simulink model "batteryModuleDoc_example"  (R2023a)
settings: Solver=ode23t  StartTime=0.0  StopTime=900  MaxStep=0.05  RelTol=1e-3  AbsTol=1e-3
InitFcn:
  | % Parameters
  | battery_vecT=[273.15, 298.15, 323.15]; % [K]
  | battery_vecAhr=5*[2.9, 4.1, 4.2];        % [Ahr]
  | battery_vecSOC=[0, .25, .75, 1];       % [-]
  | %
  | battery_V0=[3.20, 3.10, 3.14; ...
  |             3.25, 3.27, 3.30;...
  |             3.28, 3.31, 3.34;...
  |             3.33, 3.50, 3.59];         % No-load voltage, V0(SOC,T)
  | battery_R0=2*[.030, .015, .002; ...
  |             .040, .017, .008; ...
  |             .039, .012, .006; ...
  |             .027, .013, .021];         % Terminal resistance, R0(SOC,T)
  | battery_R1=[.089, .076, .010; ...
  |             .042, .022, .099; ...
  |             .019, .007, .002; ...
  |             .051, .043, .029];         % First polarization resistance, R1(SOC,T)
  | battery_Tau1=[44, 148, 235; ...
  |               93, 110, 1000; ...
  |               19, 27, 133; ...
  |               .5, 22, 3];              % First time constant, tau1(SOC,T)
  | battery_R2=[.014, .382, .407; ...
  |             .028, .006, .007; ...
  |             .014, .007, .006; ...
  |             .333, .956, .912];         % Second polarization resistance, R2(SOC,T)
  | battery_Tau2=[1, 44, 5644; ...
  |               11, 24, 506; ...
  |               2, 14, 330; ...
  |               3310, 13419, 30216];     % Second time constant, tau2(SOC,T)
  | 
  | %% Battery Module : Cell Thermal
  | battery_thermalMass=500;               % Battery cell thermal mass
  | battery_thermalK_thru=0.8;             % Battery cell through-plane thermal conductivity
  | battery_thermalK_in=20;                % Battery cell in-plane thermal conductivity
  | 
  | %% Battery Module : Module Electrical
  | battery_Np=2;
  | battery_Ns=15;
  | battery_cellH=0.65;
  | battery_cellW=0.20;
  | battery_cellT=0.02;
  | battery_extR=0.001;
  | 
  | %% Battery Module : Module Thermal
  | battery_sidesHTC=1;
  | battery_extHeat=zeros(1,battery_Np*battery_Ns);
  | 
  | %% Battery Module : Cell-to-Cell Variation
  | battery_iniT=ambientTemp*ones(1,battery_Np*battery_Ns);
  | battery_iniSOC=initialSOCvalue*ones(1,battery_Np*battery_Ns);
  | battery_varAhr=ones(1,battery_Np*battery_Ns);
  | battery_varR0=ones(1,battery_Np*battery_Ns);
  | %
  | %
  | vec_coolant_T=[295 300 305];
  | vec_coolant_F=[0.01 0.03 0.07 0.10];
  | %
  | vec_T_size=max(size(vec_coolant_T));
  | vec_F_size=max(size(vec_coolant_F));
  | mat_cellQ=zeros(vec_T_size,vec_F_size,battery_Np*battery_Ns);
  | % Inputs
  | FlwR=coolantMassFlowRate/max(vec_coolant_F);
  | FlwT=coolantTemp-ambientTemp;
undefined symbols (not defined in the file or in its folder): airGapBetweenModuleSmall, endPlateThickness
libraries: fl_lib x26, nesl_utility x6, batteryModule_lib x2
Description:
  | Battery Pack Thermal Management
  | 
  | Copyright 2020-2023 The MathWorks, Inc.
settings Model: Creator=vikrants  LastModifiedBy=smiller
settings SolverCC: AutoScaleAbsTol=off  AlgebraicLoopSolver=TrustRegion
settings DataIOCC: ReturnWorkspaceOutputs=off  SignalLoggingName=logsout_Battery_Module_To_FullPack_Grouped
settings DebuggingCC: UnconnectedInputMsg=warning  UnconnectedOutputMsg=warning  UnconnectedLineMsg=warning  SymbolicDimsDataTypeCodeGenerationDiagnostic=none
settings ModelReferenceCC: EnableRefExpFcnMdlSchedulingChecks=on
settings SFSimCC: CustomCodeUndefinedFunction=UseInterfaceOnly
settings RTWCC: DLArmComputeVersion=19.05
settings SimscapeCC: SimscapeLogType=all  SimscapeLogSimulationStatistics=on  SimscapeLogName=simlog_Battery_Module_To_FullPack_Grouped  SimscapeLogDataHistory=250000

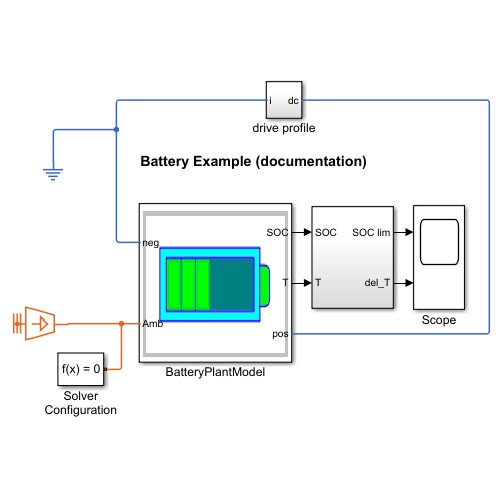
[thumbnail: Simulink's stored preview of the top-level diagram]
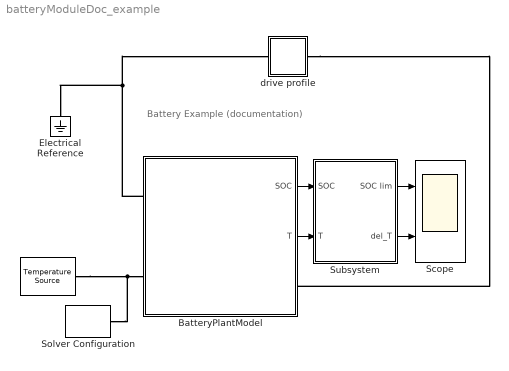
== system batteryModuleDoc_example ==
  note: Battery Example (documentation)
  " " : fl_lib/Thermal/Thermal Sources/Temperature Source  temperature=ambientTemp K
  BatteryPlantModel : Subsystem
      mask Display: image('EV_Thermal_Management_BatteryIcon.png'); % Use "Edit Image" on toolstrip to change.
  Electrical Reference : fl_lib/Electrical/Electrical Elements/Electrical Reference
  Scope : Scope  NumInputPorts=2
  Solver Configuration : nesl_utility/Solver Configuration  PhysicalDomain=network_engine_domain  SubClassName=solver  LeftPortType=input  RightPortType=generic  Tones=[]  Harmonics=[]  SimulateNoise=off  Profile=off  UseLocalSampling=off  EnableSwitchedLinearOptims=on  FrequencyDomain=off  UseCCode=off  RelTol=0.001  AbsTol=1e-06  MinStep=1e-09  ToWorkspace=off  RevertToSquareIcSolve=off  NumHomotopyIterations=100  PhasorMode=off  PhasorModeNumHarmonics=1  ConsistencySolver=NEWTON_FTOL  IndexReductionMethod=DerivativeReplacement  DoDC=off  ResidualTolerance=1e-09  ConsistencyTolSource=GLOBAL  ConsistencyAbsTol=0.001  ConsistencyRelTol=0.001  ConsistencyTolFactor=0.001  UseLocalSolver=off  LocalSolverChoice=NE_BACKWARD_EULER_ADVANCER  ResolveIndetEquations=on  FunctionEvalNumThread=1  LocalSolverSampleTime=0.001  DoFixedCost=off  MaxNonlinIter=3  MaxModeIter=2  ComputeImpulses=off  ImpulseIterations=2  LinearAlgebra=auto  LinearAlgebraNumThread=0  EquationFormulation=NE_TIME_EF  DelaysMemoryBudget=1024  AutomaticFiltering=on  FilteringTimeConstant=0.001  PartitionStorageMethod=AS_NEEDED  PartitionMemoryBudget=1024  PartitionMethod=ROBUST
  Subsystem : Subsystem
  drive profile : Subsystem
  wires:
  Subsystem/1(SOC lim) -> Scope/1
  Subsystem/2(del_T) -> Scope/2
  BatteryPlantModel/1(SOC) -> Subsystem/1(SOC)
  BatteryPlantModel/2(T) -> Subsystem/2(T)
  connections:
  " "/LConn1 -- Solver Configuration/RConn1 -- BatteryPlantModel/LConn2
  BatteryPlantModel/LConn1 -- drive profile/RConn1 -- Electrical Reference/LConn1
  drive profile/LConn1 -- BatteryPlantModel/RConn1

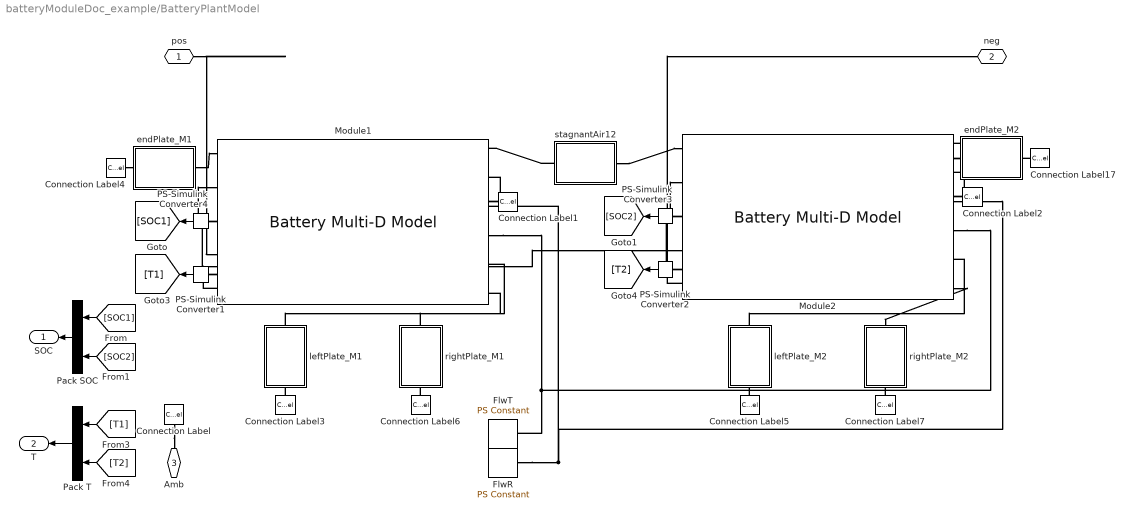
== system batteryModuleDoc_example/BatteryPlantModel ==
  Connection Label{,1..7,17} (9 alike) : ConnectionLabel  Label=amb
  FlwR : fl_lib/Physical Signals/Sources/PS Constant  constant=FlwR
  FlwT : fl_lib/Physical Signals/Sources/PS Constant  constant=FlwT K
  Module1 : batteryModule_lib/Battery Multi-D Model  modelComplexity=batteryModule.batteryAbstractionLevel.grouped  LUTpointsTemp=battery_vecT K  cellAH=4.1 A*hr  LUTpointsSOC=battery_vecSOC  V0_mat=battery_V0 V  prm_dir=ee.enum.battery.prm_dir.noCurrentDirectionality  R0_mat=battery_R0 Ohm  R0_dis_mat=[.03, .015, .002; .04, .017, .008; .039, .012, .006; .027, .013, .021] Ohm  R0_ch_mat=[.03, .015, .002; .04, .017, .008; .039, .012, .006; .027, .013, .021] Ohm  prm_leak=ee.enum.battery.prm_leak.disabled  Rleak_vec=[8000, 7000, 6000] Ohm  extrapolation_option=ee.enum.extrapolation.nearest  prm_dyn=ee.enum.battery.prm_dyn.rc2  R1_mat=battery_R1 Ohm  tau1_mat=battery_Tau1 s  R2_mat=battery_R2 Ohm  tau2_mat=battery_Tau2 s  R3_mat=[.014, .382, .407; .028, .006, .007; .014, .007, .006; .333, .956, .912] Ohm  tau3_mat=[1, 44, 5644; 11, 24, 506; 2, 14, 330; 3310, 13419, 30216] s  R4_mat=[.014, .382, .407; .028, .006, .007; .014, .007, .006; .333, .956, .912] Ohm  tau4_mat=[1, 44, 5644; 11, 24, 506; 2, 14, 330; 3310, 13419, 30216] s  R5_mat=[.014, .382, .407; .028, .006, .007; .014, .007, .006; .333, .956, .912] Ohm  tau5_mat=[1, 44, 5644; 11, 24, 506; 2, 14, 330; 3310, 13419, 30216] s  prm_fade=ee.enum.battery.prm_fade.equations  N0=100  dV0=0  dR0=0  dAH=0  dRleak=0  dR1=0  dR2=0  dR3=0  dR4=0  dR5=0  N0vec=[100, 200, 300]  Tfadevec=[298.15, 323.15] K  dV0vec=[0, 0, 0]  dR0vec=[0, 0, 0]  dAHvec=[0, 0, 0]  dRleakvec=[0, 0, 0]  dR1vec=[0, 0, 0]  dR2vec=[0, 0, 0]  dR3vec=[0, 0, 0]  dR4vec=[0, 0, 0]  dR5vec=[0, 0, 0]  dV0mat=[0, 0; 0, 0; 0, 0]  dR0mat=[0, 0; 0, 0; 0, 0]  dAHmat=[0, 0; 0, 0; 0, 0]  dRleakmat=[0, 0; 0, 0; 0, 0]  dR1mat=[0, 0; 0, 0; 0, 0]  dR2mat=[0, 0; 0, 0; 0, 0]  dR3mat=[0, 0; 0, 0; 0, 0]  dR4mat=[0, 0; 0, 0; 0, 0]  dR5mat=[0, 0; 0, 0; 0, 0]  cellThermalMass=battery_thermalMass J/K  cellThermalCond=battery_thermalK_thru W/(m*K)  cellThermalCond_inPlane=battery_thermalK_in W/(m*K)  Ns=battery_Ns  Np=battery_Np  cellTypeSelection=batteryModule.batteryTypeSelection.pouch  cellHeight=battery_cellH m  cellWidth=battery_cellW m  cellThickness=battery_cellT m  cellDiameter=0.018 m  cellCylinLine=3  moduleExternalR=battery_extR Ohm  moduleCellBalancing=batteryModule.batteryCellBalancing.none  passiveShuntR=50 Ohm  passiveSWclosedR=0.01 Ohm  passiveSWopenCond=1e-8 1/Ohm  passiveSWthreshold=0.5  moduleCellVoltages=batteryModule.batteryCellVoltages.no  thermalManagement=batteryModule.batteryCoolingSystem.thermalPort  cellHeatTrCoeff=1 W/(m^2 * K)  thermal_moduleBottom=batteryModule.batteryThermalPortSelection.thermalLUT  htc_bottom=1 W/(m^2 * K)  moduleCooling_b=mat_cellQ W/K  LUTpointsFlowrate_b=vec_coolant_F kg/s  LUTpointsTemp_b=vec_coolant_T K  thermal_moduleTop=batteryModule.batteryThermalPortSelection.convectionBC  htc_top=battery_sidesHTC W/(m^2 * K)  moduleCooling_t=zeros(3, 6, 10) W/K  LUTpointsFlowrate_t=[.01, .02, .03, .04, .05, .06] kg/s  LUTpointsTemp_t=[273.15, 298.15, 323.15] K  thermal_moduleRight=batteryModule.batteryThermalPortSelection.thermalPortLumped  htc_right=battery_sidesHTC W/(m^2 * K)  moduleCooling_r=zeros(3, 6, 10) W/K  LUTpointsFlowrate_r=[.01, .02, .03, .04, .05, .06] kg/s  LUTpointsTemp_r=[273.15, 298.15, 323.15] K  thermal_moduleLeft=batteryModule.batteryThermalPortSelection.thermalPortLumped  htc_left=battery_sidesHTC W/(m^2 * K)  moduleCooling_l=zeros(3, 6, 10) W/K  LUTpointsFlowrate_l=[.01, .02, .03, .04, .05, .06] kg/s  LUTpointsTemp_l=[273.15, 298.15, 323.15] K  thermal_modulePos=batteryModule.batteryThermalPortSelection.thermalPortLumped  htc_pos=battery_sidesHTC W/(m^2 * K)  moduleCooling_p=zeros(3, 6, 10) W/K  LUTpointsFlowrate_p=[.01, .02, .03, .04, .05, .06] kg/s  LUTpointsTemp_p=[273.15, 298.15, 323.15] K  thermal_moduleNeg=batteryModule.batteryThermalPortSelection.thermalPortLumped  htc_neg=battery_sidesHTC W/(m^2 * K)  moduleCooling_n=zeros(3, 6, 10) W/K  LUTpointsFlowrate_n=[.01, .02, .03, .04, .05, .06] kg/s  LUTpointsTemp_n=[273.15, 298.15, 323.15] K  moduleExtHeat=battery_extHeat W  cellTemp=battery_iniT K  cellSOC=battery_iniSOC  moduleCellAHpercentVar=battery_varAhr_M1  moduleCellLeakPercentVar=ones(1, 10)  moduleCellR0PercentVar=battery_varR0_M1
      settings: InternalSimscapePortConfiguration="{\"Bottom\":[{\"id\":\"Ql\",\"label\":\"Ql\",\"type\":\"foundation.thermal.thermal\"},{\"id\":\"Qr\",\"label\":\"Qr\",\"type\":\"foundation.thermal.thermal\"}],\"Left\":[{\"id\":\"Qp\",\"label\":\"Qp\",\"type\":\"foundation.thermal.thermal\"},{\"id\":\"outputCellSOC\",\"label\":\"SOC\",\"type\":\"output\"},{\"id\":\"outputCellTemp\",\"label\":\"Temp\",\"type\":\"output\"}],\"Right\":[{\"id\":\"Qn\",\"label\":\"Qn\",\"type\":\"foundation.thermal.thermal\"},{\"id\":\"H\",\"label\":\"Amb\",\"type\":\"foundation.thermal.thermal\"},{\"id\":\"frac_b\",\"label\":\"FlwR\",\"type\":\"input\"},{\"id\":\"delT_b\",\"label\":\"FlwT\",\"type\":\"input\"}],\"Top\":[{\"id\":\"p\",\"label\":\"pos\",\"type\":\"foundation.electrical.electrical\"},{\"id\":\"n\",\"label\":\"neg\",\"type\":\"foundation.electrical.electrical\"}]}"
  Module2 : batteryModule_lib/Battery Multi-D Model  modelComplexity=batteryModule.batteryAbstractionLevel.grouped  LUTpointsTemp=battery_vecT K  cellAH=4.1 A*hr  LUTpointsSOC=battery_vecSOC  V0_mat=battery_V0 V  prm_dir=ee.enum.battery.prm_dir.noCurrentDirectionality  R0_mat=battery_R0 Ohm  R0_dis_mat=[.03, .015, .002; .04, .017, .008; .039, .012, .006; .027, .013, .021] Ohm  R0_ch_mat=[.03, .015, .002; .04, .017, .008; .039, .012, .006; .027, .013, .021] Ohm  prm_leak=ee.enum.battery.prm_leak.disabled  Rleak_vec=[8000, 7000, 6000] Ohm  extrapolation_option=ee.enum.extrapolation.nearest  prm_dyn=ee.enum.battery.prm_dyn.rc2  R1_mat=battery_R1 Ohm  tau1_mat=battery_Tau1 s  R2_mat=battery_R2 Ohm  tau2_mat=battery_Tau2 s  R3_mat=[.014, .382, .407; .028, .006, .007; .014, .007, .006; .333, .956, .912] Ohm  tau3_mat=[1, 44, 5644; 11, 24, 506; 2, 14, 330; 3310, 13419, 30216] s  R4_mat=[.014, .382, .407; .028, .006, .007; .014, .007, .006; .333, .956, .912] Ohm  tau4_mat=[1, 44, 5644; 11, 24, 506; 2, 14, 330; 3310, 13419, 30216] s  R5_mat=[.014, .382, .407; .028, .006, .007; .014, .007, .006; .333, .956, .912] Ohm  tau5_mat=[1, 44, 5644; 11, 24, 506; 2, 14, 330; 3310, 13419, 30216] s  prm_fade=ee.enum.battery.prm_fade.equations  N0=100  dV0=0  dR0=0  dAH=0  dRleak=0  dR1=0  dR2=0  dR3=0  dR4=0  dR5=0  N0vec=[100, 200, 300]  Tfadevec=[298.15, 323.15] K  dV0vec=[0, 0, 0]  dR0vec=[0, 0, 0]  dAHvec=[0, 0, 0]  dRleakvec=[0, 0, 0]  dR1vec=[0, 0, 0]  dR2vec=[0, 0, 0]  dR3vec=[0, 0, 0]  dR4vec=[0, 0, 0]  dR5vec=[0, 0, 0]  dV0mat=[0, 0; 0, 0; 0, 0]  dR0mat=[0, 0; 0, 0; 0, 0]  dAHmat=[0, 0; 0, 0; 0, 0]  dRleakmat=[0, 0; 0, 0; 0, 0]  dR1mat=[0, 0; 0, 0; 0, 0]  dR2mat=[0, 0; 0, 0; 0, 0]  dR3mat=[0, 0; 0, 0; 0, 0]  dR4mat=[0, 0; 0, 0; 0, 0]  dR5mat=[0, 0; 0, 0; 0, 0]  cellThermalMass=battery_thermalMass J/K  cellThermalCond=battery_thermalK_thru W/(m*K)  cellThermalCond_inPlane=battery_thermalK_in W/(m*K)  Ns=battery_Ns  Np=battery_Np  cellTypeSelection=batteryModule.batteryTypeSelection.pouch  cellHeight=battery_cellH m  cellWidth=battery_cellW m  cellThickness=battery_cellT m  cellDiameter=0.018 m  cellCylinLine=3  moduleExternalR=battery_extR Ohm  moduleCellBalancing=batteryModule.batteryCellBalancing.none  passiveShuntR=50 Ohm  passiveSWclosedR=0.01 Ohm  passiveSWopenCond=1e-8 1/Ohm  passiveSWthreshold=0.5  moduleCellVoltages=batteryModule.batteryCellVoltages.no  thermalManagement=batteryModule.batteryCoolingSystem.thermalPort  cellHeatTrCoeff=1 W/(m^2 * K)  thermal_moduleBottom=batteryModule.batteryThermalPortSelection.thermalLUT  htc_bottom=1 W/(m^2 * K)  moduleCooling_b=mat_cellQ W/K  LUTpointsFlowrate_b=vec_coolant_F kg/s  LUTpointsTemp_b=vec_coolant_T K  thermal_moduleTop=batteryModule.batteryThermalPortSelection.convectionBC  htc_top=battery_sidesHTC W/(m^2 * K)  moduleCooling_t=zeros(3, 6, 10) W/K  LUTpointsFlowrate_t=[.01, .02, .03, .04, .05, .06] kg/s  LUTpointsTemp_t=[273.15, 298.15, 323.15] K  thermal_moduleRight=batteryModule.batteryThermalPortSelection.thermalPortLumped  htc_right=battery_sidesHTC W/(m^2 * K)  moduleCooling_r=zeros(3, 6, 10) W/K  LUTpointsFlowrate_r=[.01, .02, .03, .04, .05, .06] kg/s  LUTpointsTemp_r=[273.15, 298.15, 323.15] K  thermal_moduleLeft=batteryModule.batteryThermalPortSelection.thermalPortLumped  htc_left=battery_sidesHTC W/(m^2 * K)  moduleCooling_l=zeros(3, 6, 10) W/K  LUTpointsFlowrate_l=[.01, .02, .03, .04, .05, .06] kg/s  LUTpointsTemp_l=[273.15, 298.15, 323.15] K  thermal_modulePos=batteryModule.batteryThermalPortSelection.thermalPortLumped  htc_pos=battery_sidesHTC W/(m^2 * K)  moduleCooling_p=zeros(3, 6, 10) W/K  LUTpointsFlowrate_p=[.01, .02, .03, .04, .05, .06] kg/s  LUTpointsTemp_p=[273.15, 298.15, 323.15] K  thermal_moduleNeg=batteryModule.batteryThermalPortSelection.thermalPortLumped  htc_neg=battery_sidesHTC W/(m^2 * K)  moduleCooling_n=zeros(3, 6, 10) W/K  LUTpointsFlowrate_n=[.01, .02, .03, .04, .05, .06] kg/s  LUTpointsTemp_n=[273.15, 298.15, 323.15] K  moduleExtHeat=battery_extHeat W  cellTemp=battery_iniT K  cellSOC=battery_iniSOC  moduleCellAHpercentVar=battery_varAhr_M2  moduleCellLeakPercentVar=ones(1, 10)  moduleCellR0PercentVar=battery_varR0_M2
      settings: InternalSimscapePortConfiguration="{\"Bottom\":[{\"id\":\"Ql\",\"label\":\"Ql\",\"type\":\"foundation.thermal.thermal\"},{\"id\":\"Qr\",\"label\":\"Qr\",\"type\":\"foundation.thermal.thermal\"}],\"Left\":[{\"id\":\"Qp\",\"label\":\"Qp\",\"type\":\"foundation.thermal.thermal\"},{\"id\":\"outputCellSOC\",\"label\":\"SOC\",\"type\":\"output\"},{\"id\":\"outputCellTemp\",\"label\":\"Temp\",\"type\":\"output\"}],\"Right\":[{\"id\":\"Qn\",\"label\":\"Qn\",\"type\":\"foundation.thermal.thermal\"},{\"id\":\"H\",\"label\":\"Amb\",\"type\":\"foundation.thermal.thermal\"},{\"id\":\"frac_b\",\"label\":\"FlwR\",\"type\":\"input\"},{\"id\":\"delT_b\",\"label\":\"FlwT\",\"type\":\"input\"}],\"Top\":[{\"id\":\"p\",\"label\":\"pos\",\"type\":\"foundation.electrical.electrical\"},{\"id\":\"n\",\"label\":\"neg\",\"type\":\"foundation.electrical.electrical\"}]}"
  PS-Simulink Converter1 : nesl_utility/PS-Simulink Converter  PhysicalDomain=network_engine_domain  SubClassName=ps_output  LeftPortType=input  RightPortType=output  PseudoPeriodic=off  Frequencies=[]  VectorFormat=1-D array  Unit=K  AffineConversion=on
  PS-Simulink Converter2 : nesl_utility/PS-Simulink Converter  PhysicalDomain=network_engine_domain  SubClassName=ps_output  LeftPortType=input  RightPortType=output  PseudoPeriodic=off  Frequencies=[]  VectorFormat=1-D array  Unit=K  AffineConversion=on
  PS-Simulink Converter3 : nesl_utility/PS-Simulink Converter  PhysicalDomain=network_engine_domain  SubClassName=ps_output  LeftPortType=input  RightPortType=output  PseudoPeriodic=off  Frequencies=[]  VectorFormat=1-D array  Unit=1  AffineConversion=on
  PS-Simulink Converter4 : nesl_utility/PS-Simulink Converter  PhysicalDomain=network_engine_domain  SubClassName=ps_output  LeftPortType=input  RightPortType=output  PseudoPeriodic=off  Frequencies=[]  VectorFormat=1-D array  Unit=1  AffineConversion=on
  Pack SOC : Concatenate
  Pack T : Concatenate
  endPlate_M1 : Subsystem
  endPlate_M2 : Subsystem
  leftPlate_M1 : Subsystem
  leftPlate_M2 : Subsystem
  rightPlate_M1 : Subsystem
  rightPlate_M2 : Subsystem
  stagnantAir12 : Subsystem
  pos : PMIOPort  Side=Right
  neg : PMIOPort  Port=2  Side=Left
  Amb : PMIOPort  Port=3  Side=Left
  SOC : Outport
  T : Outport  Port=2
  wires:
  Pack SOC/1 -> SOC/1
  Pack T/1 -> T/1
  [SOC1] -> Pack SOC/1
  [SOC2] -> Pack SOC/2
  PS-Simulink Converter3/1 -> [SOC2]
  PS-Simulink Converter4/1 -> [SOC1]
  PS-Simulink Converter1/1 -> [T1]
  [T1] -> Pack T/1
  PS-Simulink Converter2/1 -> [T2]
  [T2] -> Pack T/2
  connections:
  Connection Label/LConn1 -- Amb/RConn1
  Connection Label1/LConn1 -- Module1/RConn2
  PS-Simulink Converter3/LConn1 -- Module2/LConn2
  PS-Simulink Converter2/LConn1 -- Module2/LConn3
  Connection Label2/LConn1 -- Module2/RConn2
  Module2/LConn5 -- neg/RConn1
  Module1/LConn5 -- Module2/LConn4
  pos/RConn1 -- Module1/LConn4
  PS-Simulink Converter1/LConn1 -- Module1/LConn3
  PS-Simulink Converter4/LConn1 -- Module1/LConn2
  Connection Label4/LConn1 -- endPlate_M1/LConn1
  endPlate_M1/RConn1 -- Module1/LConn1
  Connection Label17/LConn1 -- endPlate_M2/LConn1
  endPlate_M2/RConn1 -- Module2/RConn1
  rightPlate_M1/RConn1 -- Module1/RConn6
  Connection Label6/LConn1 -- rightPlate_M1/LConn1
  Connection Label3/LConn1 -- leftPlate_M1/LConn1
  leftPlate_M1/RConn1 -- Module1/RConn5
  Connection Label5/LConn1 -- leftPlate_M2/LConn1
  Connection Label7/LConn1 -- rightPlate_M2/LConn1
  Module2/RConn6 -- rightPlate_M2/RConn1
  leftPlate_M2/RConn1 -- Module2/RConn5
  stagnantAir12/LConn1 -- Module1/RConn1
  stagnantAir12/RConn1 -- Module2/LConn1
  FlwR/RConn1 -- Module2/RConn3 -- Module1/RConn3
  Module1/RConn4 -- Module2/RConn4 -- FlwT/RConn1

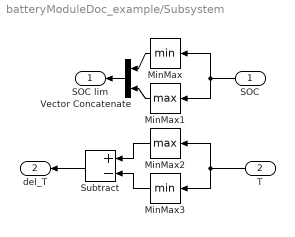
== system batteryModuleDoc_example/Subsystem ==
  SOC : Inport
  T : Inport  Port=2
  MinMax : MinMax
  MinMax1 : MinMax  Function=max
  MinMax2 : MinMax  Function=max
  MinMax3 : MinMax
  Subtract : Sum  Inputs=+-
  Vector Concatenate : Concatenate
  SOC lim : Outport
  del_T : Outport  Port=2
  wires:
  MinMax/1 -> Vector Concatenate/1
  SOC/1 -> MinMax/1, MinMax1/1
  Vector Concatenate/1 -> SOC lim/1
  MinMax1/1 -> Vector Concatenate/2
  T/1 -> MinMax2/1, MinMax3/1
  MinMax2/1 -> Subtract/1
  MinMax3/1 -> Subtract/2
  Subtract/1 -> del_T/1

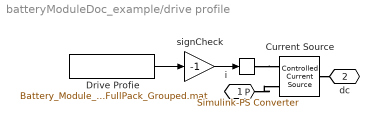
== system batteryModuleDoc_example/drive profile ==
  Current Source : fl_lib/Electrical/Electrical Sources/Controlled Current Source
  Drive Profie : FromFile  FileName=Battery_Module_To_FullPack_Grouped.mat  SampleTime=0
  P : nesl_utility/Simulink-PS Converter  PhysicalDomain=network_engine_domain  SubClassName=ps_input  LeftPortType=input  RightPortType=output  PseudoPeriodic=off  Frequencies=[]  NoiseDistribution=none  NoiseParameters=[]  Unit=A  AffineConversion=off  FilteringAndDerivatives=provide  SimscapeFilterOrder=1  InputFilterTimeConstant=0.001  UdotUserProvided=0
  signCheck : Gain  Gain=-1
  i : PMIOPort  Side=Right
  dc : PMIOPort  Port=2  Side=Left
  wires:
  Drive Profie/1 -> signCheck/1
  signCheck/1 -> P/1
  connections:
  P/RConn1 -- Current Source/RConn1
  i/RConn1 -- Current Source/RConn2
  Current Source/LConn1 -- dc/RConn1

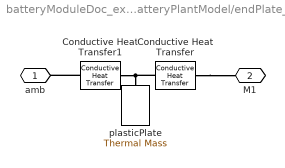
== system batteryModuleDoc_example/BatteryPlantModel/endPlate_M1 ==
  Conductive Heat Transfer : fl_lib/Thermal/Thermal Elements/Conductive Heat Transfer  thermal_type=foundation.enum.ConstantVariableTabulated.Constant  wall_geometry=foundation.enum.ConductionWallGeometry.Planar  area=battery_cellH*battery_cellW m^2  thickness=endPlateThickness m  d_in=0.05 m  d_out=0.1 m  L=1 m  th_cond_min=10 W/(K*m)  th_cond=0.024 W/(m*K)  th_cond_TLU=[413, 401, 392, 383, 371, 357, 342] W/(K*m)  temp_TLU=[200, 273, 400, 600, 800, 1000, 1200] K  T_specify=off  T_priority=None  T=0 K  T_nominal_specify=off  T_nominal_unit=K  T_nominal_value=1  Q_specify=off  Q_priority=None  Q=0 W  Q_nominal_specify=off  Q_nominal_unit=W  Q_nominal_value=1
  Conductive Heat Transfer1 : fl_lib/Thermal/Thermal Elements/Conductive Heat Transfer  thermal_type=foundation.enum.ConstantVariableTabulated.Constant  wall_geometry=foundation.enum.ConductionWallGeometry.Planar  area=battery_cellH*battery_cellW m^2  thickness=endPlateThickness m  d_in=0.05 m  d_out=0.1 m  L=1 m  th_cond_min=10 W/(K*m)  th_cond=0.024 W/(m*K)  th_cond_TLU=[413, 401, 392, 383, 371, 357, 342] W/(K*m)  temp_TLU=[200, 273, 400, 600, 800, 1000, 1200] K  T_specify=off  T_priority=None  T=0 K  T_nominal_specify=off  T_nominal_unit=K  T_nominal_value=1  Q_specify=off  Q_priority=None  Q=0 W  Q_nominal_specify=off  Q_nominal_unit=W  Q_nominal_value=1
  plasticPlate : fl_lib/Thermal/Thermal Elements/Thermal Mass  mass_type=foundation.enum.constant_variable.constant  mass=battery_cellH*battery_cellW*endPlateThickness*44 kg  sp_heat=400 J/kg/K  mass_min=1e-6 kg  num_ports=foundation.enum.numPorts2.one  m_specify=off  m_priority=High  m=1 kg  m_nominal_specify=off  m_nominal_unit=kg  m_nominal_value=1  T_specify=off  T_priority=High  T=300 K  T_nominal_specify=off  T_nominal_unit=K  T_nominal_value=1  Q_specify=off  Q_priority=None  Q=0 W  Q_nominal_specify=off  Q_nominal_unit=W  Q_nominal_value=1
  amb : PMIOPort  Side=Left
  M1 : PMIOPort  Port=2  Side=Right
  connections:
  Conductive Heat Transfer1/LConn1 -- plasticPlate/LConn1 -- Conductive Heat Transfer/RConn1
  Conductive Heat Transfer/LConn1 -- M1/RConn1
  Conductive Heat Transfer1/RConn1 -- amb/RConn1

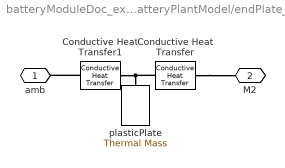
== system batteryModuleDoc_example/BatteryPlantModel/endPlate_M2 ==
  Conductive Heat Transfer : fl_lib/Thermal/Thermal Elements/Conductive Heat Transfer  thermal_type=foundation.enum.ConstantVariableTabulated.Constant  wall_geometry=foundation.enum.ConductionWallGeometry.Planar  area=battery_cellH*battery_cellW m^2  thickness=endPlateThickness m  d_in=0.05 m  d_out=0.1 m  L=1 m  th_cond_min=10 W/(K*m)  th_cond=0.024 W/(m*K)  th_cond_TLU=[413, 401, 392, 383, 371, 357, 342] W/(K*m)  temp_TLU=[200, 273, 400, 600, 800, 1000, 1200] K  T_specify=off  T_priority=None  T=0 K  T_nominal_specify=off  T_nominal_unit=K  T_nominal_value=1  Q_specify=off  Q_priority=None  Q=0 W  Q_nominal_specify=off  Q_nominal_unit=W  Q_nominal_value=1
  Conductive Heat Transfer1 : fl_lib/Thermal/Thermal Elements/Conductive Heat Transfer  thermal_type=foundation.enum.ConstantVariableTabulated.Constant  wall_geometry=foundation.enum.ConductionWallGeometry.Planar  area=battery_cellH*battery_cellW m^2  thickness=endPlateThickness m  d_in=0.05 m  d_out=0.1 m  L=1 m  th_cond_min=10 W/(K*m)  th_cond=0.024 W/(m*K)  th_cond_TLU=[413, 401, 392, 383, 371, 357, 342] W/(K*m)  temp_TLU=[200, 273, 400, 600, 800, 1000, 1200] K  T_specify=off  T_priority=None  T=0 K  T_nominal_specify=off  T_nominal_unit=K  T_nominal_value=1  Q_specify=off  Q_priority=None  Q=0 W  Q_nominal_specify=off  Q_nominal_unit=W  Q_nominal_value=1
  plasticPlate : fl_lib/Thermal/Thermal Elements/Thermal Mass  mass_type=foundation.enum.constant_variable.constant  mass=battery_cellH*battery_cellW*endPlateThickness*44 kg  sp_heat=400 J/kg/K  mass_min=1e-6 kg  num_ports=foundation.enum.numPorts2.one  m_specify=off  m_priority=High  m=1 kg  m_nominal_specify=off  m_nominal_unit=kg  m_nominal_value=1  T_specify=off  T_priority=High  T=300 K  T_nominal_specify=off  T_nominal_unit=K  T_nominal_value=1  Q_specify=off  Q_priority=None  Q=0 W  Q_nominal_specify=off  Q_nominal_unit=W  Q_nominal_value=1
  amb : PMIOPort  Side=Left
  M2 : PMIOPort  Port=2  Side=Right
  connections:
  Conductive Heat Transfer1/LConn1 -- plasticPlate/LConn1 -- Conductive Heat Transfer/RConn1
  Conductive Heat Transfer/LConn1 -- M2/RConn1
  Conductive Heat Transfer1/RConn1 -- amb/RConn1

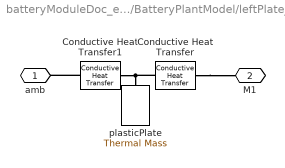
== system batteryModuleDoc_example/BatteryPlantModel/leftPlate_M1 ==
  Conductive Heat Transfer : fl_lib/Thermal/Thermal Elements/Conductive Heat Transfer  thermal_type=foundation.enum.ConstantVariableTabulated.Constant  wall_geometry=foundation.enum.ConductionWallGeometry.Planar  area=battery_cellH*battery_cellT*battery_Ns*battery_Np m^2  thickness=endPlateThickness m  d_in=0.05 m  d_out=0.1 m  L=1 m  th_cond_min=10 W/(K*m)  th_cond=0.024 W/(m*K)  th_cond_TLU=[413, 401, 392, 383, 371, 357, 342] W/(K*m)  temp_TLU=[200, 273, 400, 600, 800, 1000, 1200] K  T_specify=off  T_priority=None  T=0 K  T_nominal_specify=off  T_nominal_unit=K  T_nominal_value=1  Q_specify=off  Q_priority=None  Q=0 W  Q_nominal_specify=off  Q_nominal_unit=W  Q_nominal_value=1
  Conductive Heat Transfer1 : fl_lib/Thermal/Thermal Elements/Conductive Heat Transfer  thermal_type=foundation.enum.ConstantVariableTabulated.Constant  wall_geometry=foundation.enum.ConductionWallGeometry.Planar  area=battery_cellH*battery_cellT*battery_Ns*battery_Np m^2  thickness=endPlateThickness m  d_in=0.05 m  d_out=0.1 m  L=1 m  th_cond_min=10 W/(K*m)  th_cond=0.024 W/(m*K)  th_cond_TLU=[413, 401, 392, 383, 371, 357, 342] W/(K*m)  temp_TLU=[200, 273, 400, 600, 800, 1000, 1200] K  T_specify=off  T_priority=None  T=0 K  T_nominal_specify=off  T_nominal_unit=K  T_nominal_value=1  Q_specify=off  Q_priority=None  Q=0 W  Q_nominal_specify=off  Q_nominal_unit=W  Q_nominal_value=1
  plasticPlate : fl_lib/Thermal/Thermal Elements/Thermal Mass  mass_type=foundation.enum.constant_variable.constant  mass=battery_cellH*battery_cellT*battery_Ns*battery_Np*endPlateThickness*44 kg  sp_heat=400 J/kg/K  mass_min=1e-6 kg  num_ports=foundation.enum.numPorts2.one  m_specify=off  m_priority=High  m=1 kg  m_nominal_specify=off  m_nominal_unit=kg  m_nominal_value=1  T_specify=off  T_priority=High  T=300 K  T_nominal_specify=off  T_nominal_unit=K  T_nominal_value=1  Q_specify=off  Q_priority=None  Q=0 W  Q_nominal_specify=off  Q_nominal_unit=W  Q_nominal_value=1
  amb : PMIOPort  Side=Left
  M1 : PMIOPort  Port=2  Side=Right
  connections:
  Conductive Heat Transfer1/LConn1 -- Conductive Heat Transfer/RConn1 -- plasticPlate/LConn1
  Conductive Heat Transfer/LConn1 -- M1/RConn1
  Conductive Heat Transfer1/RConn1 -- amb/RConn1

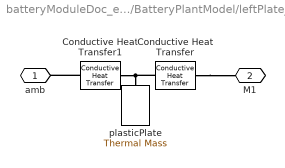
== system batteryModuleDoc_example/BatteryPlantModel/leftPlate_M2 ==
  Conductive Heat Transfer : fl_lib/Thermal/Thermal Elements/Conductive Heat Transfer  thermal_type=foundation.enum.ConstantVariableTabulated.Constant  wall_geometry=foundation.enum.ConductionWallGeometry.Planar  area=battery_cellH*battery_cellT*battery_Ns*battery_Np m^2  thickness=endPlateThickness m  d_in=0.05 m  d_out=0.1 m  L=1 m  th_cond_min=10 W/(K*m)  th_cond=0.024 W/(m*K)  th_cond_TLU=[413, 401, 392, 383, 371, 357, 342] W/(K*m)  temp_TLU=[200, 273, 400, 600, 800, 1000, 1200] K  T_specify=off  T_priority=None  T=0 K  T_nominal_specify=off  T_nominal_unit=K  T_nominal_value=1  Q_specify=off  Q_priority=None  Q=0 W  Q_nominal_specify=off  Q_nominal_unit=W  Q_nominal_value=1
  Conductive Heat Transfer1 : fl_lib/Thermal/Thermal Elements/Conductive Heat Transfer  thermal_type=foundation.enum.ConstantVariableTabulated.Constant  wall_geometry=foundation.enum.ConductionWallGeometry.Planar  area=battery_cellH*battery_cellT*battery_Ns*battery_Np m^2  thickness=endPlateThickness m  d_in=0.05 m  d_out=0.1 m  L=1 m  th_cond_min=10 W/(K*m)  th_cond=0.024 W/(m*K)  th_cond_TLU=[413, 401, 392, 383, 371, 357, 342] W/(K*m)  temp_TLU=[200, 273, 400, 600, 800, 1000, 1200] K  T_specify=off  T_priority=None  T=0 K  T_nominal_specify=off  T_nominal_unit=K  T_nominal_value=1  Q_specify=off  Q_priority=None  Q=0 W  Q_nominal_specify=off  Q_nominal_unit=W  Q_nominal_value=1
  plasticPlate : fl_lib/Thermal/Thermal Elements/Thermal Mass  mass_type=foundation.enum.constant_variable.constant  mass=battery_cellH*battery_cellT*battery_Ns*battery_Np*endPlateThickness*44 kg  sp_heat=400 J/kg/K  mass_min=1e-6 kg  num_ports=foundation.enum.numPorts2.one  m_specify=off  m_priority=High  m=1 kg  m_nominal_specify=off  m_nominal_unit=kg  m_nominal_value=1  T_specify=off  T_priority=High  T=300 K  T_nominal_specify=off  T_nominal_unit=K  T_nominal_value=1  Q_specify=off  Q_priority=None  Q=0 W  Q_nominal_specify=off  Q_nominal_unit=W  Q_nominal_value=1
  amb : PMIOPort  Side=Left
  M1 : PMIOPort  Port=2  Side=Right
  connections:
  Conductive Heat Transfer1/LConn1 -- Conductive Heat Transfer/RConn1 -- plasticPlate/LConn1
  Conductive Heat Transfer/LConn1 -- M1/RConn1
  Conductive Heat Transfer1/RConn1 -- amb/RConn1

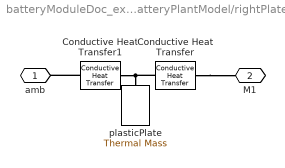
== system batteryModuleDoc_example/BatteryPlantModel/rightPlate_M1 ==
  Conductive Heat Transfer : fl_lib/Thermal/Thermal Elements/Conductive Heat Transfer  thermal_type=foundation.enum.ConstantVariableTabulated.Constant  wall_geometry=foundation.enum.ConductionWallGeometry.Planar  area=battery_cellH*battery_cellT*battery_Ns*battery_Np m^2  thickness=endPlateThickness m  d_in=0.05 m  d_out=0.1 m  L=1 m  th_cond_min=10 W/(K*m)  th_cond=0.024 W/(m*K)  th_cond_TLU=[413, 401, 392, 383, 371, 357, 342] W/(K*m)  temp_TLU=[200, 273, 400, 600, 800, 1000, 1200] K  T_specify=off  T_priority=None  T=0 K  T_nominal_specify=off  T_nominal_unit=K  T_nominal_value=1  Q_specify=off  Q_priority=None  Q=0 W  Q_nominal_specify=off  Q_nominal_unit=W  Q_nominal_value=1
  Conductive Heat Transfer1 : fl_lib/Thermal/Thermal Elements/Conductive Heat Transfer  thermal_type=foundation.enum.ConstantVariableTabulated.Constant  wall_geometry=foundation.enum.ConductionWallGeometry.Planar  area=battery_cellH*battery_cellT*battery_Ns*battery_Np m^2  thickness=endPlateThickness m  d_in=0.05 m  d_out=0.1 m  L=1 m  th_cond_min=10 W/(K*m)  th_cond=0.024 W/(m*K)  th_cond_TLU=[413, 401, 392, 383, 371, 357, 342] W/(K*m)  temp_TLU=[200, 273, 400, 600, 800, 1000, 1200] K  T_specify=off  T_priority=None  T=0 K  T_nominal_specify=off  T_nominal_unit=K  T_nominal_value=1  Q_specify=off  Q_priority=None  Q=0 W  Q_nominal_specify=off  Q_nominal_unit=W  Q_nominal_value=1
  plasticPlate : fl_lib/Thermal/Thermal Elements/Thermal Mass  mass_type=foundation.enum.constant_variable.constant  mass=battery_cellH*battery_cellT*battery_Ns*battery_Np*endPlateThickness*44 kg  sp_heat=400 J/kg/K  mass_min=1e-6 kg  num_ports=foundation.enum.numPorts2.one  m_specify=off  m_priority=High  m=1 kg  m_nominal_specify=off  m_nominal_unit=kg  m_nominal_value=1  T_specify=off  T_priority=High  T=300 K  T_nominal_specify=off  T_nominal_unit=K  T_nominal_value=1  Q_specify=off  Q_priority=None  Q=0 W  Q_nominal_specify=off  Q_nominal_unit=W  Q_nominal_value=1
  amb : PMIOPort  Side=Left
  M1 : PMIOPort  Port=2  Side=Right
  connections:
  Conductive Heat Transfer1/LConn1 -- Conductive Heat Transfer/RConn1 -- plasticPlate/LConn1
  Conductive Heat Transfer/LConn1 -- M1/RConn1
  Conductive Heat Transfer1/RConn1 -- amb/RConn1

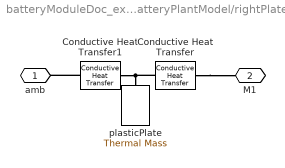
== system batteryModuleDoc_example/BatteryPlantModel/rightPlate_M2 ==
  Conductive Heat Transfer : fl_lib/Thermal/Thermal Elements/Conductive Heat Transfer  thermal_type=foundation.enum.ConstantVariableTabulated.Constant  wall_geometry=foundation.enum.ConductionWallGeometry.Planar  area=battery_cellH*battery_cellT*battery_Ns*battery_Np m^2  thickness=endPlateThickness m  d_in=0.05 m  d_out=0.1 m  L=1 m  th_cond_min=10 W/(K*m)  th_cond=0.024 W/(m*K)  th_cond_TLU=[413, 401, 392, 383, 371, 357, 342] W/(K*m)  temp_TLU=[200, 273, 400, 600, 800, 1000, 1200] K  T_specify=off  T_priority=None  T=0 K  T_nominal_specify=off  T_nominal_unit=K  T_nominal_value=1  Q_specify=off  Q_priority=None  Q=0 W  Q_nominal_specify=off  Q_nominal_unit=W  Q_nominal_value=1
  Conductive Heat Transfer1 : fl_lib/Thermal/Thermal Elements/Conductive Heat Transfer  thermal_type=foundation.enum.ConstantVariableTabulated.Constant  wall_geometry=foundation.enum.ConductionWallGeometry.Planar  area=battery_cellH*battery_cellT*battery_Ns*battery_Np m^2  thickness=endPlateThickness m  d_in=0.05 m  d_out=0.1 m  L=1 m  th_cond_min=10 W/(K*m)  th_cond=0.024 W/(m*K)  th_cond_TLU=[413, 401, 392, 383, 371, 357, 342] W/(K*m)  temp_TLU=[200, 273, 400, 600, 800, 1000, 1200] K  T_specify=off  T_priority=None  T=0 K  T_nominal_specify=off  T_nominal_unit=K  T_nominal_value=1  Q_specify=off  Q_priority=None  Q=0 W  Q_nominal_specify=off  Q_nominal_unit=W  Q_nominal_value=1
  plasticPlate : fl_lib/Thermal/Thermal Elements/Thermal Mass  mass_type=foundation.enum.constant_variable.constant  mass=battery_cellH*battery_cellT*battery_Ns*battery_Np*endPlateThickness*44 kg  sp_heat=400 J/kg/K  mass_min=1e-6 kg  num_ports=foundation.enum.numPorts2.one  m_specify=off  m_priority=High  m=1 kg  m_nominal_specify=off  m_nominal_unit=kg  m_nominal_value=1  T_specify=off  T_priority=High  T=300 K  T_nominal_specify=off  T_nominal_unit=K  T_nominal_value=1  Q_specify=off  Q_priority=None  Q=0 W  Q_nominal_specify=off  Q_nominal_unit=W  Q_nominal_value=1
  amb : PMIOPort  Side=Left
  M1 : PMIOPort  Port=2  Side=Right
  connections:
  Conductive Heat Transfer1/LConn1 -- Conductive Heat Transfer/RConn1 -- plasticPlate/LConn1
  Conductive Heat Transfer/LConn1 -- M1/RConn1
  Conductive Heat Transfer1/RConn1 -- amb/RConn1

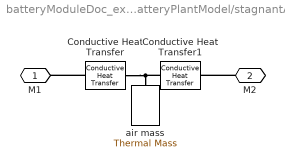
== system batteryModuleDoc_example/BatteryPlantModel/stagnantAir12 ==
  Conductive Heat Transfer : fl_lib/Thermal/Thermal Elements/Conductive Heat Transfer  thermal_type=foundation.enum.ConstantVariableTabulated.Constant  wall_geometry=foundation.enum.ConductionWallGeometry.Planar  area=battery_cellH*battery_cellW m^2  thickness=airGapBetweenModuleSmall m  d_in=0.05 m  d_out=0.1 m  L=1 m  th_cond_min=10 W/(K*m)  th_cond=0.024 W/(m*K)  th_cond_TLU=[413, 401, 392, 383, 371, 357, 342] W/(K*m)  temp_TLU=[200, 273, 400, 600, 800, 1000, 1200] K  T_specify=off  T_priority=None  T=0 K  T_nominal_specify=off  T_nominal_unit=K  T_nominal_value=1  Q_specify=off  Q_priority=None  Q=0 W  Q_nominal_specify=off  Q_nominal_unit=W  Q_nominal_value=1
  Conductive Heat Transfer1 : fl_lib/Thermal/Thermal Elements/Conductive Heat Transfer  thermal_type=foundation.enum.ConstantVariableTabulated.Constant  wall_geometry=foundation.enum.ConductionWallGeometry.Planar  area=battery_cellH*battery_cellW m^2  thickness=airGapBetweenModuleSmall m  d_in=0.05 m  d_out=0.1 m  L=1 m  th_cond_min=10 W/(K*m)  th_cond=0.024 W/(m*K)  th_cond_TLU=[413, 401, 392, 383, 371, 357, 342] W/(K*m)  temp_TLU=[200, 273, 400, 600, 800, 1000, 1200] K  T_specify=off  T_priority=None  T=0 K  T_nominal_specify=off  T_nominal_unit=K  T_nominal_value=1  Q_specify=off  Q_priority=None  Q=0 W  Q_nominal_specify=off  Q_nominal_unit=W  Q_nominal_value=1
  air mass : fl_lib/Thermal/Thermal Elements/Thermal Mass  mass_type=foundation.enum.constant_variable.constant  mass=battery_cellH*battery_cellW*airGapBetweenModuleSmall*1.28 kg  sp_heat=1000 J/kg/K  mass_min=1e-6 kg  num_ports=foundation.enum.numPorts2.one  m_specify=off  m_priority=High  m=1 kg  m_nominal_specify=off  m_nominal_unit=kg  m_nominal_value=1  T_specify=off  T_priority=High  T=300 K  T_nominal_specify=off  T_nominal_unit=K  T_nominal_value=1  Q_specify=off  Q_priority=None  Q=0 W  Q_nominal_specify=off  Q_nominal_unit=W  Q_nominal_value=1
  M1 : PMIOPort  Side=Left
  M2 : PMIOPort  Port=2  Side=Right
  connections:
  Conductive Heat Transfer/LConn1 -- M1/RConn1
  M2/RConn1 -- Conductive Heat Transfer1/RConn1
  Conductive Heat Transfer1/LConn1 -- air mass/LConn1 -- Conductive Heat Transfer/RConn1
